simulink model "Part1_3_a"  (R2019a)
settings: Solver=VariableStepAuto  StartTime=0.0  StopTime=103  RelTol=1e-3
libraries: simulink x1
settings Model: Creator=admin  LastModifiedBy=admin

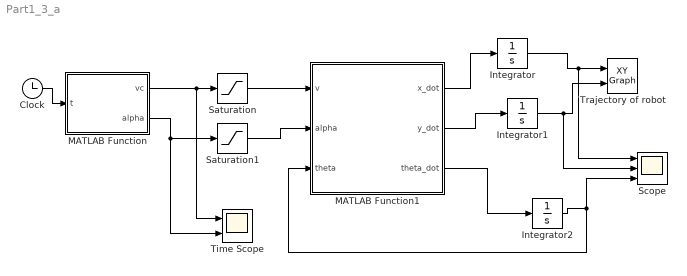
== system Part1_3_a ==
  Clock : Clock
      settings: Decimation=100
  Integrator : Integrator
  Integrator1 : Integrator
  Integrator2 : Integrator
  MATLAB Function : MATLAB Function  TreatAsAtomicUnit=on
  MATLAB Function1 : MATLAB Function  TreatAsAtomicUnit=on
  Saturation : Saturate  UpperLimit=1.8  LowerLimit=-1.8
  Saturation1 : Saturate  UpperLimit=pi/4  LowerLimit=-pi/4
  Scope : Scope  NumInputPorts=3
  Time Scope : Scope  NumInputPorts=2
  Trajectory of robot : simulink/Sinks/XY Graph  xmin=-30  xmax=50  ymin=-30  ymax=30  st=-1
  wires:
  MATLAB Function/2(alpha) -> Time Scope/2, Saturation1/1
  Saturation1/1 -> MATLAB Function1/2(alpha)
  Integrator/1 -> Trajectory of robot/1, Scope/1
  Integrator2/1 -> MATLAB Function1/3(theta), Scope/3
  MATLAB Function1/3(theta_dot) -> Integrator2/1
  MATLAB Function1/2(y_dot) -> Integrator1/1
  MATLAB Function/1(vc) -> Time Scope/1, Saturation/1
  MATLAB Function1/1(x_dot) -> Integrator/1
  Integrator1/1 -> Scope/2, Trajectory of robot/2
  Saturation/1 -> MATLAB Function1/1(v)
  Clock/1 -> MATLAB Function/1(t)

== matlab function Part1_3_a/MATLAB Function1 ==
  data: v input; x_dot output; alpha input; theta input; y_dot output; theta_dot output
function [x_dot, y_dot, theta_dot] = tricycle_type_2(v, alpha, theta)

d = sqrt(3.1);
x_dot = v*cos(theta);
y_dot = v*sin(theta);
theta_dot = v/d*tan(alpha);

== matlab function Part1_3_a/MATLAB Function ==
  data: t input; vc output; alpha output
function [vc, alpha] = input(t)
if t < 20
    vc = 1;
    alpha = 0;
elseif t <= 20 + pi/0.05
    vc = 0.2;
    alpha = -atan(0.05*sqrt(3.1)/vc);
else 
    vc = 1;
    alpha = 0;
end
end
